simulink model "scheme"  (R2025b)
settings: Solver=VariableStepAuto  StartTime=0.0  StopTime=20.0  RelTol=1e-3
settings Model: Creator=Teacher  LastModifiedBy=pc
settings SolverCC: AlgebraicLoopSolver=TrustRegion
settings DebuggingCC: UnconnectedInputMsg=warning  UnconnectedOutputMsg=warning  UnconnectedLineMsg=warning
settings ModelReferenceCC: EnableRefExpFcnMdlSchedulingChecks=on
settings RTWCC: GPUComputeCapability=3.5

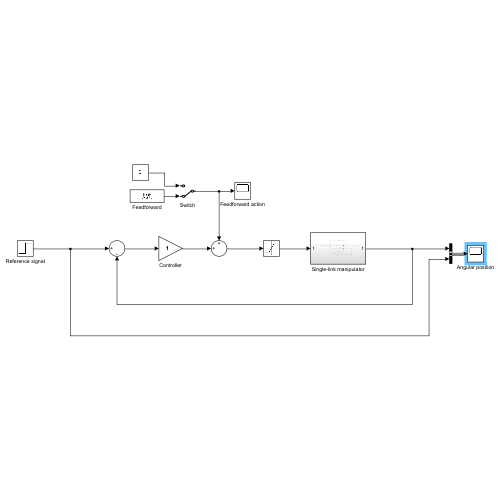
[thumbnail: Simulink's stored preview of the top-level diagram]
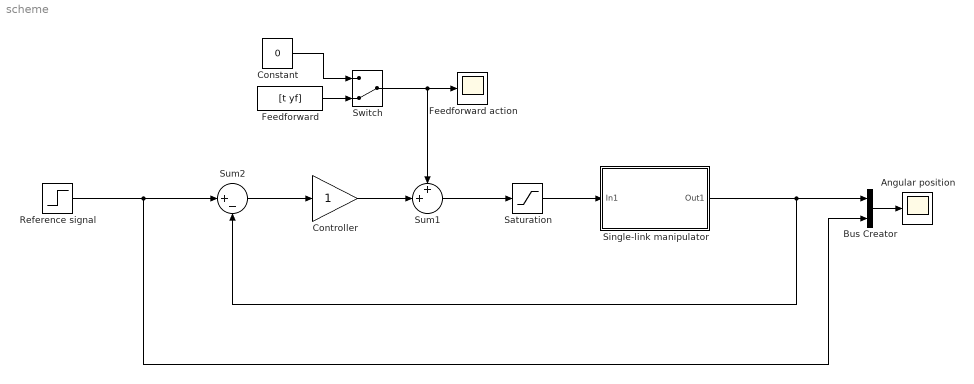
== system scheme ==
  Angular position : Scope
      settings: ActiveDisplayYMinimum=-5.1376060099772332  ActiveDisplayYMaximum=14.690069282975152
  Bus Creator : BusCreator  Inputs=2
  Constant : Constant  Value=0
  Controller : Gain
  Feedforward : FromWorkspace  VariableName=[t yf]
  Feedforward action : Scope
      settings: ActiveDisplayYMinimum=-1.22324  ActiveDisplayYMaximum=6.26117  DataLoggingVariableName=ScopeData2
  Reference signal : Step  After=10  SampleTime=0
  Saturation : Saturate  UpperLimit=10  LowerLimit=-10
  Single-link manipulator : Subsystem
  Sum1 : Sum  Inputs=++|
  Sum2 : Sum  Inputs=|+-
  Switch : ManualSwitch  CurrentSetting=0
  wires:
  Sum2/1 -> Controller/1
  Controller/1 -> Sum1/2
  Sum1/1 -> Saturation/1
  Switch/1 -> Feedforward action/1, Sum1/1
  Constant/1 -> Switch/1
  Feedforward/1 -> Switch/2
  Reference signal/1 -> Bus Creator/2, Sum2/1
  Single-link manipulator/1(Out1) -> Sum2/2, Bus Creator/1
  Saturation/1 -> Single-link manipulator/1(In1)
  Bus Creator/1 -> Angular position/1

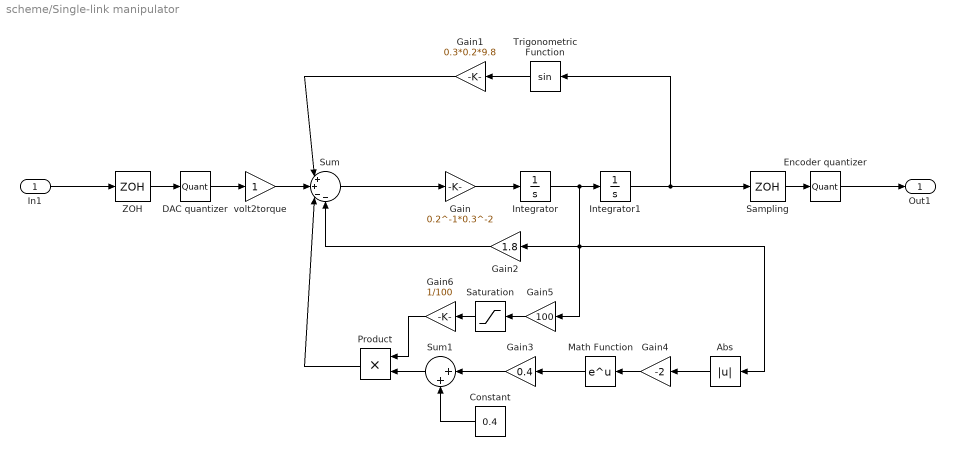
== system scheme/Single-link manipulator ==
  In1 : Inport
  Abs : Abs  SaturateOnIntegerOverflow=off
  Constant : Constant  Value=0.4
  DAC quantizer : Quantizer  QuantizationInterval=10/2^13
  Encoder quantizer : Quantizer  QuantizationInterval=2*pi/3000
  Gain : Gain  Gain=0.2^-1*0.3^-2
  Gain1 : Gain  Gain=0.3*0.2*9.8
  Gain2 : Gain  Gain=1.8
  Gain3 : Gain  Gain=0.4
  Gain4 : Gain  Gain=-2
  Gain5 : Gain  Gain=100
  Gain6 : Gain  Gain=1/100
  Integrator : Integrator
  Integrator1 : Integrator
  Math Function : Math
  Product : Product
  Sampling : ZeroOrderHold  SampleTime=0.001
  Saturation : Saturate  UpperLimit=1  LowerLimit=-1
  Sum : Sum  Inputs=|++--
  Sum1 : Sum  Inputs=|++
  Trigonometric Function : Trigonometry
  ZOH : ZeroOrderHold  SampleTime=0.001
  volt2torque : Gain
  Out1 : Outport
  wires:
  Gain/1 -> Integrator/1
  Gain3/1 -> Sum1/1
  Sum1/1 -> Product/2
  Gain6/1 -> Product/1
  Gain5/1 -> Saturation/1
  Gain2/1 -> Sum/4
  Gain1/1 -> Sum/1
  Integrator1/1 -> Sampling/1, Trigonometric Function/1
  Saturation/1 -> Gain6/1
  Trigonometric Function/1 -> Gain1/1
  Product/1 -> Sum/3
  Sum/1 -> Gain/1
  Constant/1 -> Sum1/2
  Integrator/1 -> Gain5/1, Abs/1, Gain2/1, Integrator1/1
  Abs/1 -> Gain4/1
  Gain4/1 -> Math Function/1
  Math Function/1 -> Gain3/1
  Sampling/1 -> Encoder quantizer/1
  Encoder quantizer/1 -> Out1/1
  ZOH/1 -> DAC quantizer/1
  DAC quantizer/1 -> volt2torque/1
  volt2torque/1 -> Sum/2
  In1/1 -> ZOH/1
